simulink model "Am"  (R2022b)
settings: Solver=FixedStepAuto  StartTime=0.0  StopTime=22  FixedStep=1/44100  RelTol=1e-3
settings Model: Creator=mirab  LastModifiedBy=mirab

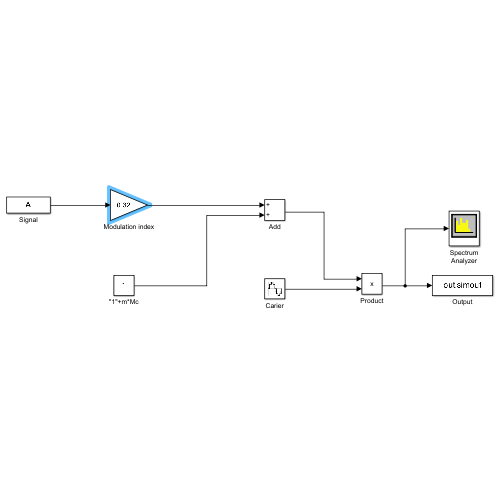
[thumbnail: Simulink's stored preview of the top-level diagram]
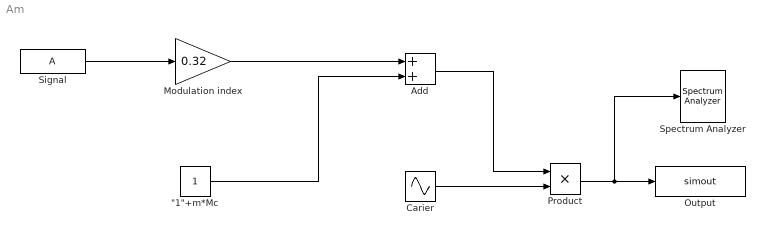
== system Am ==
  "\"1\"+m*Mc" : Constant
  Add : Sum
  Carier : Sin  Frequency=1000000  SampleTime=1/44100
  Modulation index : Gain  Gain=0.32
  Output : ToWorkspace  VariableName=simout  SaveFormat=Timeseries  SampleTime=-1
  Product : Product
  Signal : FromWorkspace  VariableName=A  SampleTime=1/44100
  Spectrum Analyzer : SpectrumAnalyzer
  wires:
  Modulation index/1 -> Add/1
  Add/1 -> Product/1
  "\"1\"+m*Mc"/1 -> Add/2
  Carier/1 -> Product/2
  Signal/1 -> Modulation index/1
  Product/1 -> Spectrum Analyzer/1, Output/1
